simulink model "c2000_top_model_pil"  (R2021b)
settings: Solver=FixedStepDiscrete  StartTime=0.0  StopTime=10.0  FixedStep=T  RelTol=1e-3  EnableMultiTasking=on
PostLoadFcn:
  | % Ensure the Simulation Data Inspector is opened automatically
  | % set_param(gcs, 'InspectSignalLogs', 'on');
  | 
  | % Sample time
  | T=0.1;
  | [ticks_to_count, reset, counter_mode, count_enable, ...
  |         counter_mode_values_run1, counter_mode_values_run2, ...
  |         count_enable_values_run1, count_enable_values_run2] = ...
  |     tic2000_pil_topmodel_data(T);
  | 
  | % Parameters
  | countUpper = uint8(40);
  | countLower = uint8(20);
  | counter_mode_select = 0;
  | %Signals
  | enableA = mpt.Signal;
  | enableA.CoderInfo.CustomStorageClass = 'FileScope';
  | enableB = mpt.Signal;
  | enableB.CoderInfo.CustomStorageClass = 'FileScope';
InitFcn:
  | % Ensure the Simulation Data Inspector is opened automatically
  | % set_param(gcs, 'InspectSignalLogs', 'on');
  | 
  | % Sample time
  | T=0.1;
  | [ticks_to_count, reset, counter_mode, count_enable, ...
  |         counter_mode_values_run1, counter_mode_values_run2, ...
  |         count_enable_values_run1, count_enable_values_run2] = ...
  |     tic2000_pil_topmodel_data(T);
  | 
  | % Parameters
  | countUpper = uint8(40);
  | countLower = uint8(20);
  | counter_mode_select = 0;
  | %Signals
  | enableA = mpt.Signal;
  | enableA.CoderInfo.CustomStorageClass = 'FileScope';
  | enableB = mpt.Signal;
  | enableB.CoderInfo.CustomStorageClass = 'FileScope';
Description:
  | Example model reference component.
settings Model: FPTRunName=Active  SimulationMode=processor-in-the-loop (pil)  CodeVerificationMode=processor-in-the-loop (pil)  ExtModeTrigDuration=8  Creator=The MathWorks, Inc.  LastModifiedBy=The MathWorks, Inc.
settings SolverCC: AlgebraicLoopSolver=TrustRegion
settings DataIOCC: ExternalInput=ticks_to_count, reset, counter_mode, count_enable  LoadExternalInput=on  SaveFormat=StructureWithTime  SaveOutput=off  DSMLogging=off  SaveTime=off  ReturnWorkspaceOutputs=off  SignalLoggingName=logsOut
settings OptimizationCC: UseDivisionForNetSlopeComputation=UseDivisionForReciprocalsOfIntegersOnly  EnhancedBackFolding=on  BooleansAsBitfields=on  PassReuseOutputArgsAs=Individual arguments  ExpressionDepthLimit=2147483647  StateBitsets=on  DataBitsets=on  NoFixptDivByZeroProtection=on  EfficientFloat2IntCast=on  LifeSpan=1  MaxStackSize=512  SimCompilerOptimization=on  DenormalBehavior=FlushToZero  EfficientTunableParamExpr=on
settings DebuggingCC: ReadBeforeWriteMsg=DisableAll  WriteAfterWriteMsg=DisableAll  WriteAfterReadMsg=DisableAll  CheckExecutionContextPreStartOutputMsg=on  FcnCallInpInsideContextMsg=warning  UniqueDataStoreMsg=error  AllowSymbolicDim=off  ModelReferenceSymbolNameMessage=none  StateNameClashWarn=warning  StrictBusMsg=ErrorOnBusTreatedAsVector  SFUnexpectedBacktrackingDiag=warning  SFNoUnconditionalDefaultTransitionDiag=warning  SFExecutionAtInitializationDiag=none  SFMachineParentedDataDiag=warning  ArithmeticOperatorsInVariantConditions=warning
settings HardwareCC: ProdBitPerChar=16  ProdBitPerInt=16  ProdBitPerPointer=32  ProdBitPerSizeT=32  ProdBitPerPtrDiffT=32  ProdLargestAtomicInteger=Integer  ProdLargestAtomicFloat=None  ProdWordSize=16  ProdLongLongMode=on  ProdHWDeviceType=Texas Instruments->C2000  TargetHWDeviceType=Generic->32-bit Embedded Processor
settings ModelReferenceCC: CheckModelReferenceTargetMessage=none  ModelReferencePassRootInputsByReference=off  PropagateSignalLabelsOutOfModel=off
settings SFSimCC: SimUseLocalCustomCode=off  MATLABDynamicMemAlloc=off
settings RTWCC: Description=Embedded Coder  SystemTargetFile=ert.tlc  HardwareBoard=TI Piccolo F2806x  TemplateMakefile=ert_default_tmf  GenerateReport=on  RTWVerbose=off  RTWUseLocalCustomCode=off  Toolchain=Texas Instruments Code Composer Studio (C2000)  IncludeHyperlinkInReport=on  CodeExecutionProfiling=on  CodeProfilingSaveOptions=AllData  GenerateTraceInfo=on  GenerateTraceReport=on  GenerateTraceReportSl=on  GenerateTraceReportSf=on  GenerateTraceReportEml=on
settings CodeAppCC: ForceParamTrailComments=on  IgnoreCustomStorageClasses=off  SimulinkDataObjDesc=on  CustomSymbolStrGlobalVar=rt$N$M  CustomSymbolStrType=$N$M  CustomSymbolStrFcn=$N$M$F  CustomSymbolStrMacro=$N$M  InsertBlockDesc=on  StateflowObjectComments=on  InternalIdentifier=Classic
settings ERTTargetCC: CodeReplacementLibrary=TI C28x  UtilityFuncGeneration=Shared location  MultiwordLength=2048  IncludeMdlTerminateFcn=off  CombineSignalStateStructs=on  SupportNonFinite=off  SupportComplex=off  ExtModeStaticAllocSize=2048  ERTFilePackagingFormat=CompactWithDataFile  ConvertIfToSwitch=off  SuppressUnreachableDefaultCases=off
settings ConfigComp: CovEnable=on  CovScope=ReferencedModels  RecordCoverage=on  CovCompData=covCumulativeData  CovMetricSettings=dcmrsw  CovHTMLOptions=-aTS=1 -bRG=1 -bTC=1 -hTR=0 -nFC=0 -scm=1 -bcm=1 -xEv=0  CovSaveCumulativeToWorkspaceVar=on  CovSaveSingleToWorkspaceVar=on  CovCumulativeReport=on  CovModelRefEnable=Off  CovExternalEMLEnable=off  CovSFcnEnable=off

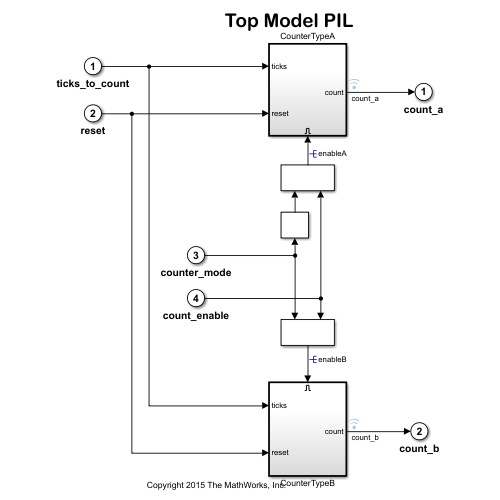
[thumbnail: Simulink's stored preview of the top-level diagram]
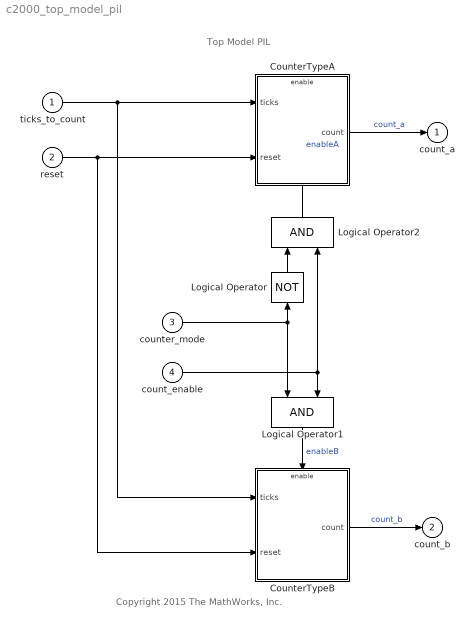
== system c2000_top_model_pil ==
  note: Copyright 2015 The MathWorks, Inc.
  note: Top Model PIL
  ticks_to_count : Inport  OutDataTypeStr=boolean  PortDimensions=1  SampleTime=T
  reset : Inport  Port=2  OutDataTypeStr=boolean  PortDimensions=1  SampleTime=T
  counter_mode : Inport  Port=3  OutDataTypeStr=boolean  PortDimensions=1  SampleTime=T
  count_enable : Inport  Port=4  OutDataTypeStr=boolean  PortDimensions=1  SampleTime=T
  CounterTypeA : Subsystem
      settings: RTWSystemCode=Nonreusable function  RTWFcnNameOpts=Use subsystem name
  CounterTypeB : Subsystem
      settings: RTWSystemCode=Nonreusable function  RTWFcnNameOpts=Use subsystem name
  Logical Operator : Logic  Operator=NOT  AllPortsSameDT=off  OutDataTypeStr=boolean
  Logical Operator1 : Logic  AllPortsSameDT=off  OutDataTypeStr=boolean
  Logical Operator2 : Logic  AllPortsSameDT=off  OutDataTypeStr=boolean
  count_a : Outport  VectorParamsAs1DForOutWhenUnconnected=off
  count_b : Outport  Port=2  VectorParamsAs1DForOutWhenUnconnected=off
  wires:
  ticks_to_count/1 -> CounterTypeA/1(ticks), CounterTypeB/1(ticks)
  reset/1 -> CounterTypeA/2(reset), CounterTypeB/2(reset)
  CounterTypeA/1(count) -> count_a/1  "count_a"
  CounterTypeB/1(count) -> count_b/1  "count_b"
  Logical Operator1/1 -> CounterTypeB/Enable  "enableB"
  Logical Operator2/1 -> CounterTypeA/Enable  "enableA"
  Logical Operator/1 -> Logical Operator2/1
  counter_mode/1 -> Logical Operator1/1, Logical Operator/1
  count_enable/1 -> Logical Operator1/2, Logical Operator2/2

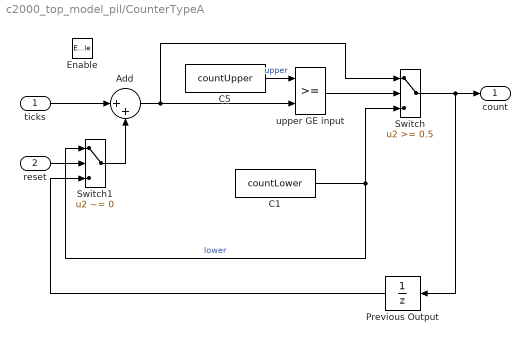
== system c2000_top_model_pil/CounterTypeA ==
  ticks : Inport
  reset : Inport  Port=2
  Enable : EnablePort
  Add : Sum  Inputs=|++  OutDataTypeStr=uint8
  C1 : Constant  Value=countLower  OutDataTypeStr=uint8
  C5 : Constant  Value=countUpper  OutDataTypeStr=uint8
  Previous Output : UnitDelay  InitialCondition=25  SampleTime=T  HasFrameUpgradeWarning=on
  Switch : Switch  Threshold=0.5  InputSameDT=on
  Switch1 : Switch  Criteria=u2 ~= 0  Threshold=0.5  InputSameDT=on
  upper GE input : RelationalOperator  Priority=0  OutDataTypeStr=boolean  RndMeth=Nearest  InputSameDT=on
      settings: AttributesFormatString=\n
  count : Outport  InitialOutput=25  VectorParamsAs1DForOutWhenUnconnected=off
  wires:
  Switch/1 -> Previous Output/1, count/1
  upper GE input/1 -> Switch/2
  C5/1 -> upper GE input/1  "upper"
  Add/1 -> upper GE input/2, Switch/1
  C1/1 -> Switch/3, Switch1/1  "lower"
  Previous Output/1 -> Switch1/3
  Switch1/1 -> Add/2
  ticks/1 -> Add/1
  reset/1 -> Switch1/2

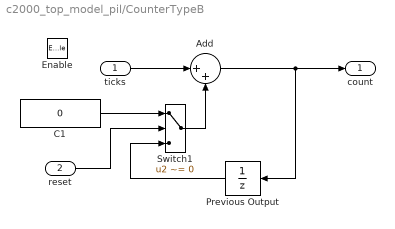
== system c2000_top_model_pil/CounterTypeB ==
  ticks : Inport
  reset : Inport  Port=2
  Enable : EnablePort
  Add : Sum  Inputs=|++  OutDataTypeStr=uint8
  C1 : Constant  Value=0  OutDataTypeStr=uint8
  Previous Output : UnitDelay  InitialCondition=15  SampleTime=T  HasFrameUpgradeWarning=on
  Switch1 : Switch  Criteria=u2 ~= 0  Threshold=0.5  InputSameDT=on
  count : Outport  InitialOutput=15  VectorParamsAs1DForOutWhenUnconnected=off
  wires:
  ticks/1 -> Add/1
  reset/1 -> Switch1/2
  Switch1/1 -> Add/2
  Previous Output/1 -> Switch1/3
  Add/1 -> count/1, Previous Output/1
  C1/1 -> Switch1/1
